simulink model "doc_design_iteration_basic"  (R2014a)
settings: Solver=FixedStepDiscrete  StartTime=0.0  StopTime=inf  RelTol=1e-3
PreLoadFcn:
  | EbNo=0;
  | maxNumErrs=200;
  | maxNumBits=1e8;
libraries: commdigbbndpm3 x2, commchan3 x1, commrandsrc2 x1, commsink2 x1
Description:
  | Parallel Concatenated Convolutional Coding: Turbo Codes
  | 
  | This demo model shows the layout of the Turbo Encoder as specified by 3GPP TS 36.212 v9.0
  | and the corresponding iterative Turbo Decoder.
  | 
  | The model can be configured to run with any one of the 188 block sizes supported by the standard
  | and is set to evaluate the BER performance of the code over an AWGN channel.
settings Model: FPTRunName=Active  Creator=The MathWorks Inc.
settings DataIOCC: SaveOutput=off  DSMLogging=off  SaveTime=off
settings OptimizationCC: ExpressionDepthLimit=2147483647  RollThreshold=2  SimCompilerOptimization=On
settings DebuggingCC: UnderspecifiedInitializationDetection=Classic  StateNameClashWarn=warning
settings GRTTargetCC: CombineOutputUpdateFcns=off  GRTInterface=on

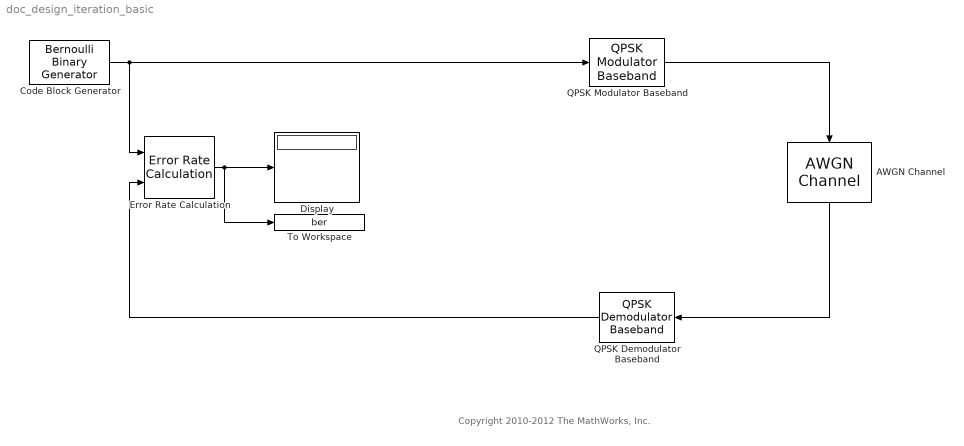
== system doc_design_iteration_basic ==
  note: Copyright 2010-2012 The MathWorks, Inc.
  AWGN Channel : commchan3/AWGN Channel  InputProcessing=Columns as channels (frame based)  seed=67  noiseMode=Variance from mask  EbNodB=10  EsNodB=10  SNRdB=10  bitsPerSym=2  Ps=1  Tsym=1  variance=10.^(-0.1*(EbNo + 10*log10(1) + 10*log10(2)))
  Code Block Generator : commrandsrc2/Bernoulli Binary Generator  P=0.5  seed=12345  Ts=1/2040  frameBased=on  sampPerFrame=2040  orient=off  outDataType=boolean
  Display : Display
  Error Rate Calculation : commsink2/Error Rate Calculation  N=0  st_delay=0  cp_mode=Entire frame  subframe=[]  PMode=Port  WsName=ErrorVec1  RsMode2=off  stop=on  numErr=maxNumErrs  maxBits=maxNumBits
  QPSK Demodulator Baseband : commdigbbndpm3/QPSK Demodulator Baseband  Ph=pi/4  Dec=Gray  OutType=Bit  DecType=Hard decision  VarSource=Dialog  Variance=1  outDtype1=boolean  outDtype2=Inherit via internal rule  derotateFactorWordLen=16
  QPSK Modulator Baseband : commdigbbndpm3/QPSK Modulator Baseband  InType=Bit  Enc=Gray  Ph=pi/4  outDtype=double  outWordLen=16  outUDDataType=sfix(16)  outFracLenMode=Best precision  outFracLen=15
  To Workspace : ToWorkspace  VariableName=ber  SampleTime=-1
      settings: MaxDataPoints=1
  wires:
  Code Block Generator/1 -> Error Rate Calculation/1, QPSK Modulator Baseband/1
  AWGN Channel/1 -> QPSK Demodulator Baseband/1
  Error Rate Calculation/1 -> Display/1, To Workspace/1
  QPSK Modulator Baseband/1 -> AWGN Channel/1
  QPSK Demodulator Baseband/1 -> Error Rate Calculation/2
